simulink model "S_Mod_Sim_PV_V1"  (R2017a)
settings: Solver=VariableStepAuto  StartTime=0.0  StopTime=1.3  FixedStep=1e-6  MaxStep=1e-4  RelTol=1e-3
values from neighbouring files (symbols this model uses):
  Cdc = 470e-6    (= 0.00047)    [M_Mod_Sim_PV_V1.m]
  Cin = 1e-6    (= 1e-06)    [M_Mod_Sim_PV_V1.m]
  dIL = (vpv/L)*d*Ts1    (= 0.460350492963)    [M_Mod_Sim_PV_V1.m]
  Fred = fs    (= 60)    [M_Mod_Sim_PV_V1.m]
  fs = 60    [M_Mod_Sim_PV_V1.m]
  Icc_calc = In/(5/100)    [M_Mod_Sim_PV_V1.m]
  Kf1 = Scala/dDmax    (= 5.88235294118)    [M_Mod_Sim_PV_V1.m]
  ki = 1/ipv    (= 0.0636345580933)    [M_Mod_Sim_PV_V1.m]
  KI2 = Ki2*Ts4    [M_Mod_Sim_PV_V1.m]
  KI4 = Ki4*Ts4    [M_Mod_Sim_PV_V1.m]
  KI5 = Ki5*Ts_inv    (= 0.0710611516878)    [M_Mod_Sim_PV_V1.m]
  KP2 = Kp2 - KI2/2    [M_Mod_Sim_PV_V1.m]
  KP4 = Kp4 - KI4/2    [M_Mod_Sim_PV_V1.m]
  KP5 = Kp5*Ts_inv - KI5/2    (= -0.0349975104025)    [M_Mod_Sim_PV_V1.m]
  L = 68.2729*Lmin    (= 0.100000049318)    [M_Mod_Sim_PV_V1.m]
  Linv = 0.035    [M_Mod_Sim_PV_V1.m]
  Rinv = 0.0417    [M_Mod_Sim_PV_V1.m]
  S = 10e3*3/2    (= 15000)    [M_Mod_Sim_PV_V1.m]
  Ts1 = 1/Fs    (= 0.0002)    [M_Mod_Sim_PV_V1.m]
  Ts3 = Ts1    (= 0.0002)    [M_Mod_Sim_PV_V1.m]
  Ts4 = 1/(4*Fc)    (= 5e-05)    [M_Mod_Sim_PV_V1.m]
  Ts_inv = 1/(100*Fc)    (= 2e-06)    [M_Mod_Sim_PV_V1.m]
  vdc = 1000    [M_Mod_Sim_PV_V1.m]
  vdc_ref = vdc    (= 1000)    [M_Mod_Sim_PV_V1.m]
  Vf = VL/sqrt(3)    [M_Mod_Sim_PV_V1.m]
  VL = (381.051/2)    (= 190.5255)    [M_Mod_Sim_PV_V1.m]
undefined symbols (not defined in the file or in its folder): DiscIntNeverNeededParam
undefined symbols (not defined in the file): Fs
libraries: powerlib x15, powerlib_meascontrol x12, fuzblock x3, dsparch4 x3, re_lib x1
settings Model: Creator=dricl  LastModifiedBy=dricl

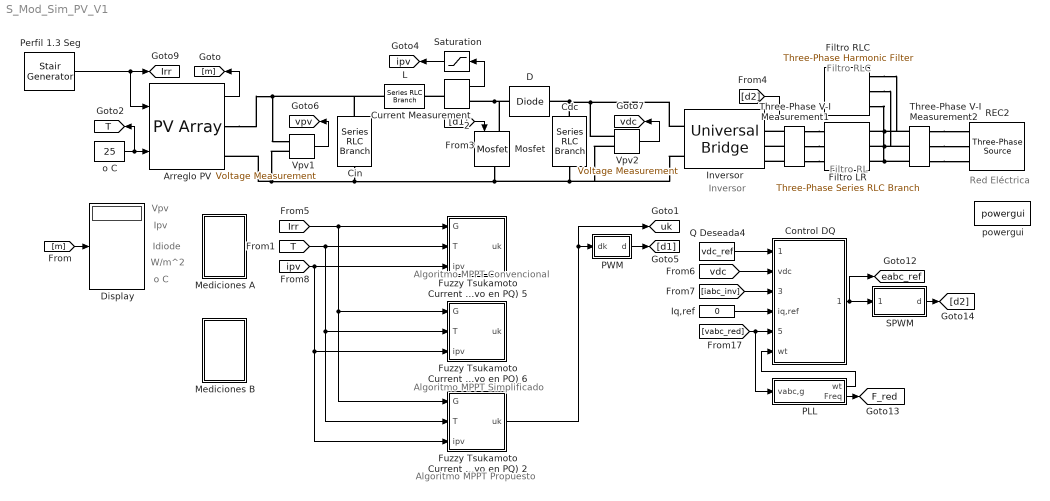
== system S_Mod_Sim_PV_V1 ==
  note: o C
  note: Idiode
  note: Ipv
  note: Vpv
  note: W/m^2
  note: Red Eléctrica
  note: Filtro RL
  note: Inversor
  note: Filtro RLC
  note: Algoritmo MPPT Convencional
  note: Algoritmo MPPT Simplificado
  note: Algoritmo MPPT Propuesto
  " Control DQ" : Subsystem
  Arreglo PV : re_lib/Solar/PV Array  Npar=No_Cadenas_Paralelo  Nser=No_Modulos_PorCadena  PlotType=array @ 1000 W/m2 & specified temperatures  S_vec=[ 1250 1000 100 ]  Temp_C_vec="[ 45 25  0]"  ModuleName=Canadian Solar CS6X-280P  PlotWhenSelected=off  Pm=279.816  Ncell=72  Voc=44.2  Isc=8.42  Vm=35.6  Im=7.86  beta_Voc_pc=-0.39  alpha_Isc_pc=0.06  beta_Voc=-0.17238  alpha_Isc=0.005052  IL=8.4417  I0=7.7188e-10  nI=1.0345  Rsh=300.2269  Rs=0.38773  BAL=off  Tc=1e-6  Tfilter=5e-5
  Cdc : powerlib/Elements/Series RLC Branch  LConnTagsString=__new0  RConnTagsString=__new0  BranchType=C  Resistance=0.01  Inductance=1e-3  SetiL0=off  InitialCurrent=0  Capacitance=Cdc  Setx0=on  InitialVoltage=vdc_ref  Measurements=None
  Cin : powerlib/Elements/Series RLC Branch  LConnTagsString=__new0  RConnTagsString=__new0  BranchType=C  Resistance=0.01  Inductance=1e-3  SetiL0=off  InitialCurrent=0  Capacitance=Cin  Setx0=off  InitialVoltage=640.8  Measurements=None
  Current Measurement2 : powerlib/Measurements/Current Measurement  PhasorSimulation=off  OutputType=Complex  PSBequivalent=0
  D : powerlib/Power Electronics/Diode  Ron=0.001  Lon=0  Vf=0  IC=0  UseSnubber=0  Rs=500  Cs=250e-9  Measurements=off
  Display : Display
  Filtro LR : powerlib/Elements/Three-Phase Series RLC Branch  LConnTagsString=A|B|C  RConnTagsString=A|B|C  BranchType=RL  Resistance=Rinv  Inductance=Linv  Capacitance=1e-6  Measurements=None
  Filtro RLC : powerlib/Elements/Three-Phase Harmonic Filter  LConnTagsString=A|B|C  FilterType=Single-tuned  FilterConnection=Y (grounded)  ParNom=[VL fs]  Qc=S*0.001  Fr=[31.42*60]  Frd=[40*fs 80*fs]  Q=5  Measurements=None
      settings: AttributesFormatString=\n  SourceProductName=Simscape Power Systems  SourceProductBaseCode=PS
  "Fuzzy Tsukamoto Current Controller n_mppt = 99.11%, ta(2%) = 0.12 s con Steps de Irrad Interv. 2 Seg. n_mppt = 96.74%, ta(2%) = 0.12 s con Steps de Irrad Interv. 0.5 Seg. n_mppt = 99.37%, ta(2%) = 0.12 s con Curva de Irrad Este controlador puede disminuir ta e incrementar a tr para mitigar los MP en id (impacto positivo en PQ) 2" : Subsystem
  "Fuzzy Tsukamoto Current Controller n_mppt = 99.11%, ta(2%) = 0.12 s con Steps de Irrad Interv. 2 Seg. n_mppt = 96.74%, ta(2%) = 0.12 s con Steps de Irrad Interv. 0.5 Seg. n_mppt = 99.37%, ta(2%) = 0.12 s con Curva de Irrad Este controlador puede disminuir ta e incrementar a tr para mitigar los MP en id (impacto positivo en PQ) 5" : Subsystem
  "Fuzzy Tsukamoto Current Controller n_mppt = 99.11%, ta(2%) = 0.12 s con Steps de Irrad Interv. 2 Seg. n_mppt = 96.74%, ta(2%) = 0.12 s con Steps de Irrad Interv. 0.5 Seg. n_mppt = 99.37%, ta(2%) = 0.12 s con Curva de Irrad Este controlador puede disminuir ta e incrementar a tr para mitigar los MP en id (impacto positivo en PQ) 6" : Subsystem
  Inversor : powerlib/Power Electronics/Universal Bridge  Arms=3  SnubberResistance=1e5  SnubberCapacitance=inf  Device=IGBT / Diodes  Ron=1e-3  Lon=0  ForwardVoltages="[  0  0  ]"  ForwardVoltage=0  GTOparameters=[ 10e-6 , 20e-6 ]  IGBTparameters=[ 1e-6 , 2e-6 ]  Measurements=None  Measurements_2=None  converterType=Rectifier
  Iq,ref : Constant  Value=0  SampleTime=Ts4
  L : powerlib/Elements/Series RLC Branch  LConnTagsString=__new0  RConnTagsString=__new0  BranchType=L  Resistance=40.76340  Inductance=L  SetiL0=off  InitialCurrent=0  Capacitance=1e-6  Setx0=off  InitialVoltage=0  Measurements=None
  Mediciones A : Subsystem
  Mediciones B : Subsystem
  Mosfet : powerlib/Power Electronics/Mosfet  Ron=0.001  Lon=0  Rd=0  Vfd=0  IC=0  Rs=1e5  Cs=inf  Measurements=off
  PLL : Subsystem
  PWM : Subsystem  AncestorBlock=plecslib_extras2/Modulators/Symmetrical PWM  mask(Symmetrical PWM){sampling=Natural (carrier starts with 0), fc=Fs, offset=0, input_limits=[0 Kf1], output_values=[0 1]}
      mask prompts: fc "Carrier frequency (Hz):"; offset "Carrier offset (p.u.):"; input_limits "Input limits [min max]:"; output_values "Output values [off on]:"
      mask help: PWM generator with a symmetrical triangular carrier. If the input is a vector, the output is also a vector of the same width.
      mask init:
      | if numel(fc)>1 || fc<=0,
      |   error('Carrier frequency must be a positive scalar.');
      | end
      | if numel(offset)>1 || offset<0 || offset>=1,
      |   error('Carrier offset must be a scalar in the range [0; 1/fc[.');
      | end
      | if sampling == 1,
      |   offset = mod(offset+.75, 1);
      | end
      | 
      | si = [.5 mod(offset, .5)]/fc;
      mask Help: eval('plecs(''help'', ''symmetricalpwm.html'')')
      mask TypeOptions sampling: Natural (carrier starts with 0) | Natural (carrier starts with 1) | Regular (double edge) | Regular (single edge)
  Perfil 1.3 Seg : powerlib_meascontrol/Pulse & Signal Generators/Stair Generator  t=[0, 0.1, 0.3, 0.5, 0.7, 0.9, 1.1]  e=[0, 1000, 400, 800, 500, 900, 600]  Ts=0
      settings: SourceProductName=Simscape Power Systems
  Q Deseada4 : Constant  Value=vdc_ref  SampleTime=Ts4
  REC2 : powerlib/Electrical Sources/Three-Phase Source  InternalConnection=Yg  VoltagePhases=on  Voltage=VL  PhaseAngle=0  Voltage_phases=[VL/sqrt(3) VL/sqrt(3) VL/sqrt(3)]  PhaseAngles_phases=[0 -120 +120]  Frequency=Fred  NonIdealSource=on  SpecifyImpedance=on  Resistance=25e3^2/10e6/5  Inductance=25e3^2/10e6/377  ShortCircuitLevel=Icc_calc*2  BaseVoltage=VL  XRratio=7  BusType=swing  Pref=-500e3  Qref=0  Prefabc=[10e3, 10e3, 10e3]  Qrefabc=[0, 0, 0]  Qmin=-inf  Qmax=inf
  SPWM : Subsystem
  Saturation : Saturate  UpperLimit=inf  LowerLimit=0
  Three-Phase V-I Measurement1 : powerlib/Measurements/Three-Phase V-I Measurement  VoltageMeasurement=phase-to-ground  SetLabelV=on  LabelV=vabc_inv  Vpu=off  VpuLL=off  CurrentMeasurement=yes  SetLabelI=on  LabelI=iabc_inv  Ipu=off  Pbase=100e6  Vbase=500e3  OutputType=Complex  PhasorSimulation=off  PSBequivalent=0
  Three-Phase V-I Measurement2 : powerlib/Measurements/Three-Phase V-I Measurement  VoltageMeasurement=phase-to-ground  SetLabelV=on  LabelV=vabc_red  Vpu=off  VpuLL=off  CurrentMeasurement=yes  SetLabelI=on  LabelI=iabc_red  Ipu=off  Pbase=100e6  Vbase=500e3  OutputType=Complex  PhasorSimulation=off  PSBequivalent=0
  Vpv1 : powerlib/Measurements/Voltage Measurement  PhasorSimulation=off  OutputType=Complex  PSBequivalent=0
  Vpv2 : powerlib/Measurements/Voltage Measurement  PhasorSimulation=off  OutputType=Complex  PSBequivalent=0
  o C : Constant  Value=25
  powergui : powerlib/powergui  Priority=1  SimulationMode=Continuous  SampleTime=1e-6  frequency=60  Iterations=50  frequencyindice=0  Pbase=100e6  ErrMax=1e-4  UnitsV=kV  UnitsW=MW  buscounter=0  FunctionMessages=off  echomessages=off  EnableUseOfTLC=off  CurrentSourceSwitches=off  DisableSnubberDevices=off  DisableRonSwitches=off  DisableVfSwitches=off  DisplayEquations=off  SolverType=Tustin/Backward Euler (TBE)  Interpol=off  ExternalGateDelay=off  methode=off  Ts=100  x0status=blocks  SPID=on  SwTol=0  HookPort=off  RestoreLinks=warning  ResistiveCurrentMeasurement=off  Frange=[0:2:500]  Ylog=off  Xlog=on  ShowGrid=off  save=off  variable=ZData  structure=logsout  ZoomFFT=on  StartTime=0.1  cycles=4  DisplayStyle=1  fundamental=60  FreqAxis=off  MaxFrequency=1000  frequencyindicesteady=1  RmsSteady=1  display=off
  tag scope: F_red=global, Irr=global, T=global, eabc_ref=global, ipv=global, uk=global, vdc=global, vpv=global
  wires:
  o C/1 -> [T], Arreglo PV/2
  Arreglo PV/1 -> [m]
  [m] -> Display/1
  Current Measurement2/1 -> Saturation/1
  Vpv1/1 -> [vpv]
  Vpv2/1 -> [vdc]
  [d1] -> Mosfet/1
  [d2] -> Inversor/1
  [vabc_red] -> " Control DQ"/5(vabc,red), PLL/1(vabc,g)
  PLL/1(wt) -> " Control DQ"/6(wt)
  [iabc_inv] -> " Control DQ"/3(iabc,inv)
  " Control DQ"/1(eabc,ref) -> [eabc_ref], SPWM/1(eabc,ref)
  PLL/2(Freq) -> [F_red]
  Iq,ref/1 -> " Control DQ"/4(iq,ref)
  [vdc] -> " Control DQ"/2(vdc)
  SPWM/1(d) -> [d2]
  PWM/1(d) -> [d1]
  Saturation/1 -> [ipv]
  Q Deseada4/1 -> " Control DQ"/1(vdc,ref)
  Perfil 1.3 Seg/1 -> Arreglo PV/1, [Irr]
  [Irr] -> "Fuzzy Tsukamoto Current Controller n_mppt = 99.11%, ta(2%) = 0.12 s con Steps de Irrad Interv. 2 Seg. n_mppt = 96.74%, ta(2%) = 0.12 s con Steps de Irrad Interv. 0.5 Seg. n_mppt = 99.37%, ta(2%) = 0.12 s con Curva de Irrad Este controlador puede disminuir ta e incrementar a tr para mitigar los MP en id (impacto positivo en PQ) 2"/1(G), "Fuzzy Tsukamoto Current Controller n_mppt = 99.11%, ta(2%) = 0.12 s con Steps de Irrad Interv. 2 Seg. n_mppt = 96.74%, ta(2%) = 0.12 s con Steps de Irrad Interv. 0.5 Seg. n_mppt = 99.37%, ta(2%) = 0.12 s con Curva de Irrad Este controlador puede disminuir ta e incrementar a tr para mitigar los MP en id (impacto positivo en PQ) 6"/1(G), "Fuzzy Tsukamoto Current Controller n_mppt = 99.11%, ta(2%) = 0.12 s con Steps de Irrad Interv. 2 Seg. n_mppt = 96.74%, ta(2%) = 0.12 s con Steps de Irrad Interv. 0.5 Seg. n_mppt = 99.37%, ta(2%) = 0.12 s con Curva de Irrad Este controlador puede disminuir ta e incrementar a tr para mitigar los MP en id (impacto positivo en PQ) 5"/1(G)
  [ipv] -> "Fuzzy Tsukamoto Current Controller n_mppt = 99.11%, ta(2%) = 0.12 s con Steps de Irrad Interv. 2 Seg. n_mppt = 96.74%, ta(2%) = 0.12 s con Steps de Irrad Interv. 0.5 Seg. n_mppt = 99.37%, ta(2%) = 0.12 s con Curva de Irrad Este controlador puede disminuir ta e incrementar a tr para mitigar los MP en id (impacto positivo en PQ) 5"/3(ipv), "Fuzzy Tsukamoto Current Controller n_mppt = 99.11%, ta(2%) = 0.12 s con Steps de Irrad Interv. 2 Seg. n_mppt = 96.74%, ta(2%) = 0.12 s con Steps de Irrad Interv. 0.5 Seg. n_mppt = 99.37%, ta(2%) = 0.12 s con Curva de Irrad Este controlador puede disminuir ta e incrementar a tr para mitigar los MP en id (impacto positivo en PQ) 2"/3(ipv), "Fuzzy Tsukamoto Current Controller n_mppt = 99.11%, ta(2%) = 0.12 s con Steps de Irrad Interv. 2 Seg. n_mppt = 96.74%, ta(2%) = 0.12 s con Steps de Irrad Interv. 0.5 Seg. n_mppt = 99.37%, ta(2%) = 0.12 s con Curva de Irrad Este controlador puede disminuir ta e incrementar a tr para mitigar los MP en id (impacto positivo en PQ) 6"/3(ipv)
  [T] -> "Fuzzy Tsukamoto Current Controller n_mppt = 99.11%, ta(2%) = 0.12 s con Steps de Irrad Interv. 2 Seg. n_mppt = 96.74%, ta(2%) = 0.12 s con Steps de Irrad Interv. 0.5 Seg. n_mppt = 99.37%, ta(2%) = 0.12 s con Curva de Irrad Este controlador puede disminuir ta e incrementar a tr para mitigar los MP en id (impacto positivo en PQ) 2"/2(T), "Fuzzy Tsukamoto Current Controller n_mppt = 99.11%, ta(2%) = 0.12 s con Steps de Irrad Interv. 2 Seg. n_mppt = 96.74%, ta(2%) = 0.12 s con Steps de Irrad Interv. 0.5 Seg. n_mppt = 99.37%, ta(2%) = 0.12 s con Curva de Irrad Este controlador puede disminuir ta e incrementar a tr para mitigar los MP en id (impacto positivo en PQ) 6"/2(T), "Fuzzy Tsukamoto Current Controller n_mppt = 99.11%, ta(2%) = 0.12 s con Steps de Irrad Interv. 2 Seg. n_mppt = 96.74%, ta(2%) = 0.12 s con Steps de Irrad Interv. 0.5 Seg. n_mppt = 99.37%, ta(2%) = 0.12 s con Curva de Irrad Este controlador puede disminuir ta e incrementar a tr para mitigar los MP en id (impacto positivo en PQ) 5"/2(T)
  "Fuzzy Tsukamoto Current Controller n_mppt = 99.11%, ta(2%) = 0.12 s con Steps de Irrad Interv. 2 Seg. n_mppt = 96.74%, ta(2%) = 0.12 s con Steps de Irrad Interv. 0.5 Seg. n_mppt = 99.37%, ta(2%) = 0.12 s con Curva de Irrad Este controlador puede disminuir ta e incrementar a tr para mitigar los MP en id (impacto positivo en PQ) 2"/1(uk) -> [uk], PWM/1(dk)
  connections:
  Arreglo PV/RConn1 -- Cin/LConn1 -- L/LConn1 -- Vpv1/LConn1
  Current Measurement2/LConn1 -- L/RConn1
  Mosfet/LConn1 -- D/LConn1 -- Current Measurement2/RConn1
  Vpv2/LConn1 -- Inversor/RConn1 -- Cdc/LConn1 -- D/RConn1
  Vpv1/LConn2 -- Cin/RConn1 -- Vpv2/LConn2 -- Inversor/RConn2 -- Cdc/RConn1 -- Mosfet/RConn1 -- Arreglo PV/RConn2
  Three-Phase V-I Measurement2/RConn1 -- REC2/RConn1
  Three-Phase V-I Measurement2/RConn2 -- REC2/RConn2
  Three-Phase V-I Measurement2/RConn3 -- REC2/RConn3
  Filtro LR/RConn2 -- Three-Phase V-I Measurement2/LConn2 -- Filtro RLC/LConn2
  Filtro LR/RConn3 -- Three-Phase V-I Measurement2/LConn3 -- Filtro RLC/LConn3
  Filtro LR/RConn1 -- Three-Phase V-I Measurement2/LConn1 -- Filtro RLC/LConn1
  Three-Phase V-I Measurement1/RConn1 -- Filtro LR/LConn1
  Three-Phase V-I Measurement1/LConn1 -- Inversor/LConn1
  Three-Phase V-I Measurement1/RConn3 -- Filtro LR/LConn3
  Three-Phase V-I Measurement1/LConn3 -- Inversor/LConn3
  Three-Phase V-I Measurement1/RConn2 -- Filtro LR/LConn2
  Three-Phase V-I Measurement1/LConn2 -- Inversor/LConn2

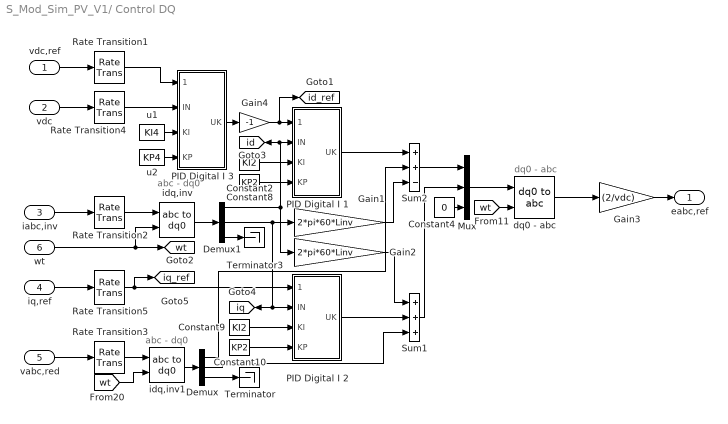
== system S_Mod_Sim_PV_V1/ Control DQ ==
  note: dq0 - abc
  note: abc - dq0
  note: abc - dq0
  vdc,ref : Inport
  vdc : Inport  Port=2
  iabc,inv : Inport  Port=3
  iq,ref : Inport  Port=4
  vabc,red : Inport  Port=5
  wt : Inport  Port=6
  Constant10 : Constant  Value=KP2  SampleTime=Ts4
  Constant2 : Constant  Value=KI2  SampleTime=Ts4
  Constant4 : Constant  Value=0  SampleTime=Ts4
  Constant8 : Constant  Value=KP2  SampleTime=Ts4
  Constant9 : Constant  Value=KI2  SampleTime=Ts4
  Demux : Demux  Outputs=3
  Demux1 : Demux  Outputs=3
  Gain1 : Gain  Gain=2*pi*60*Linv
  Gain2 : Gain  Gain=2*pi*60*Linv
  Gain3 : Gain  Gain=(2/vdc)
  Gain4 : Gain  Gain=-1
  Mux : Mux  Inputs=3
  PID Digital I 1 : MATLAB Function  TreatAsAtomicUnit=on
  PID Digital I 2 : MATLAB Function  TreatAsAtomicUnit=on
  PID Digital I 3 : MATLAB Function  TreatAsAtomicUnit=on
  Rate Transition{1..5} (5 alike) : RateTransition  OutPortSampleTime=Ts4
  Sum1 : Sum  Inputs=+++
  Sum2 : Sum  Inputs=++-
  Terminator : Terminator
  Terminator3 : Terminator
  dq0 - abc : powerlib_meascontrol/Transformations/dq0 to abc  Alignment=90 degrees behind phase A axis
  idq,inv : powerlib_meascontrol/Transformations/abc to dq0  Alignment=90 degrees behind phase A axis
  idq,inv1 : powerlib_meascontrol/Transformations/abc to dq0  Alignment=90 degrees behind phase A axis
  u1 : Constant  Value=KI4  SampleTime=Ts4
  u2 : Constant  Value=KP4  SampleTime=Ts4
  eabc,ref : Outport
  tag scope: id=global, id_ref=global, iq=global, iq_ref=global, wt=global
  wires:
  vabc,red/1 -> Rate Transition3/1
  Rate Transition4/1 -> PID Digital I 3/2(IN)
  Demux/2 -> Sum1/3
  Demux1/2 -> PID Digital I 2/2(IN), [iq], Gain1/1
  PID Digital I 1/1(UK) -> Sum2/1
  Gain4/1 -> [id_ref], PID Digital I 1/1(IN_ref)
  Sum1/1 -> Mux/2
  Mux/1 -> dq0 - abc/1
  Constant4/1 -> Mux/3
  [wt] -> dq0 - abc/2
  Demux/3 -> Terminator/1
  Demux1/1 -> [id], PID Digital I 1/2(IN), Gain2/1
  Constant8/1 -> PID Digital I 1/4(KP)
  Rate Transition5/1 -> [iq_ref], PID Digital I 2/1(IN_ref)
  idq,inv1/1 -> Demux/1
  iq,ref/1 -> Rate Transition5/1
  idq,inv/1 -> Demux1/1
  Constant9/1 -> PID Digital I 2/3(KI)
  u1/1 -> PID Digital I 3/3(KI)
  vdc,ref/1 -> Rate Transition1/1
  Constant10/1 -> PID Digital I 2/4(KP)
  vdc/1 -> Rate Transition4/1
  Constant2/1 -> PID Digital I 1/3(KI)
  iabc,inv/1 -> Rate Transition2/1
  Rate Transition2/1 -> idq,inv/1
  Demux1/3 -> Terminator3/1
  Rate Transition3/1 -> idq,inv1/1
  u2/1 -> PID Digital I 3/4(KP)
  PID Digital I 2/1(UK) -> Sum1/2
  Sum2/1 -> Mux/1
  Demux/1 -> Sum2/2
  Gain2/1 -> Sum1/1
  Gain1/1 -> Sum2/3
  [wt] -> idq,inv1/2
  wt/1 -> [wt], idq,inv/2
  dq0 - abc/1 -> Gain3/1
  PID Digital I 3/1(UK) -> Gain4/1
  Rate Transition1/1 -> PID Digital I 3/1(IN_ref)
  Gain3/1 -> eabc,ref/1

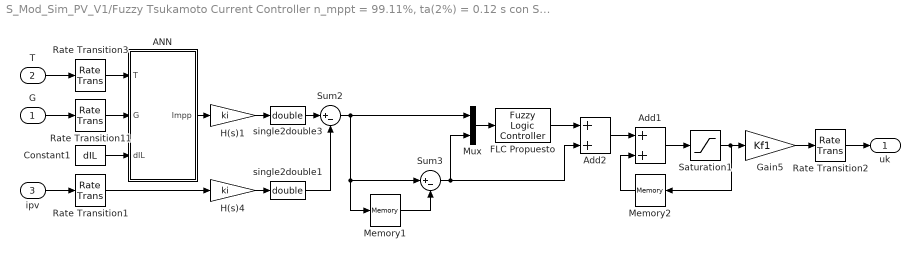
== system S_Mod_Sim_PV_V1/Fuzzy Tsukamoto Current Controller n_mppt = 99.11%, ta(2%) = 0.12 s con Steps de Irrad Interv. 2 Seg. n_mppt = 96.74%, ta(2%) = 0.12 s con Steps de Irrad Interv. 0.5 Seg. n_mppt = 99.37%, ta(2%) = 0.12 s con Curva de Irrad Este controlador puede disminuir ta e incrementar a tr para mitigar los MP en id (impacto positivo en PQ) 2 ==
  G : Inport
  T : Inport  Port=2
  ipv : Inport  Port=3
  ANN : MATLAB Function  TreatAsAtomicUnit=on
  Add1 : Sum
  Add2 : Sum
  Constant1 : Constant  Value=dIL  SampleTime=Ts3
  FLC Propuesto : fuzblock/Fuzzy Logic  Controller  fis=['5_Rules_MaMPPTCtrl_V1.fis']
  Gain5 : Gain  Gain=Kf1
  H(s)1 : Gain  Gain=ki
  H(s)4 : Gain  Gain=ki
  Memory1 : Memory  InheritSampleTime=on
  Memory2 : Memory  InheritSampleTime=on
  Mux : Mux  Inputs=2
  Rate Transition{1..3,11} (4 alike) : RateTransition  Deterministic=off  OutPortSampleTime=Ts3
  Saturation1 : Saturate  UpperLimit=1  LowerLimit=0
  Sum2 : Sum  Inputs=|+-
  Sum3 : Sum  Inputs=|+-
  single2double1 : DataTypeConversion  OutDataTypeStr=double
  single2double3 : DataTypeConversion  OutDataTypeStr=double
  uk : Outport
  wires:
  Rate Transition2/1 -> uk/1
  Memory2/1 -> Add1/2
  single2double3/1 -> Sum2/1
  single2double1/1 -> Sum2/2
  Memory1/1 -> Sum3/2
  Add1/1 -> Saturation1/1
  Saturation1/1 -> Memory2/1, Gain5/1
  Gain5/1 -> Rate Transition2/1
  H(s)1/1 -> single2double3/1
  H(s)4/1 -> single2double1/1
  ANN/1(Impp) -> H(s)1/1
  Mux/1 -> FLC Propuesto/1
  Sum2/1 -> Memory1/1, Sum3/1, Mux/1
  Sum3/1 -> Add2/2, Mux/2
  FLC Propuesto/1 -> Add2/1
  Add2/1 -> Add1/1
  G/1 -> Rate Transition11/1
  ipv/1 -> Rate Transition1/1
  Rate Transition1/1 -> H(s)4/1
  Rate Transition3/1 -> ANN/1(T)
  Rate Transition11/1 -> ANN/2(G)
  Constant1/1 -> ANN/3(dIL)
  T/1 -> Rate Transition3/1

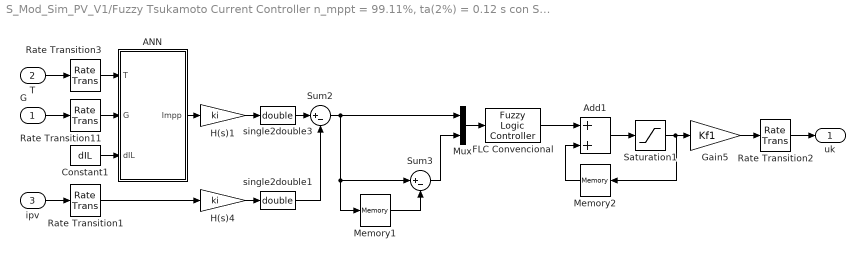
== system S_Mod_Sim_PV_V1/Fuzzy Tsukamoto Current Controller n_mppt = 99.11%, ta(2%) = 0.12 s con Steps de Irrad Interv. 2 Seg. n_mppt = 96.74%, ta(2%) = 0.12 s con Steps de Irrad Interv. 0.5 Seg. n_mppt = 99.37%, ta(2%) = 0.12 s con Curva de Irrad Este controlador puede disminuir ta e incrementar a tr para mitigar los MP en id (impacto positivo en PQ) 5 ==
  G : Inport
  T : Inport  Port=2
  ipv : Inport  Port=3
  ANN : MATLAB Function  TreatAsAtomicUnit=on
  Add1 : Sum
  Constant1 : Constant  Value=dIL  SampleTime=Ts3
  FLC Convencional : fuzblock/Fuzzy Logic  Controller  fis=['49_Rules_MaMPPTCtrlPaperShaikRAfi_V2.fis']
  Gain5 : Gain  Gain=Kf1
  H(s)1 : Gain  Gain=ki
  H(s)4 : Gain  Gain=ki
  Memory1 : Memory  InheritSampleTime=on
  Memory2 : Memory  InheritSampleTime=on
  Mux : Mux  Inputs=2
  Rate Transition{1..3,11} (4 alike) : RateTransition  Deterministic=off  OutPortSampleTime=Ts3
  Saturation1 : Saturate  UpperLimit=1  LowerLimit=0
  Sum2 : Sum  Inputs=|+-
  Sum3 : Sum  Inputs=|+-
  single2double1 : DataTypeConversion  OutDataTypeStr=double
  single2double3 : DataTypeConversion  OutDataTypeStr=double
  uk : Outport
  wires:
  Rate Transition2/1 -> uk/1
  Memory2/1 -> Add1/2
  single2double3/1 -> Sum2/1
  single2double1/1 -> Sum2/2
  Rate Transition1/1 -> H(s)4/1
  G/1 -> Rate Transition11/1
  ipv/1 -> Rate Transition1/1
  Memory1/1 -> Sum3/2
  Add1/1 -> Saturation1/1
  Saturation1/1 -> Memory2/1, Gain5/1
  Gain5/1 -> Rate Transition2/1
  H(s)1/1 -> single2double3/1
  H(s)4/1 -> single2double1/1
  ANN/1(Impp) -> H(s)1/1
  Constant1/1 -> ANN/3(dIL)
  Mux/1 -> FLC Convencional/1
  Sum2/1 -> Memory1/1, Sum3/1, Mux/1
  Sum3/1 -> Mux/2
  FLC Convencional/1 -> Add1/1
  Rate Transition11/1 -> ANN/2(G)
  Rate Transition3/1 -> ANN/1(T)
  T/1 -> Rate Transition3/1

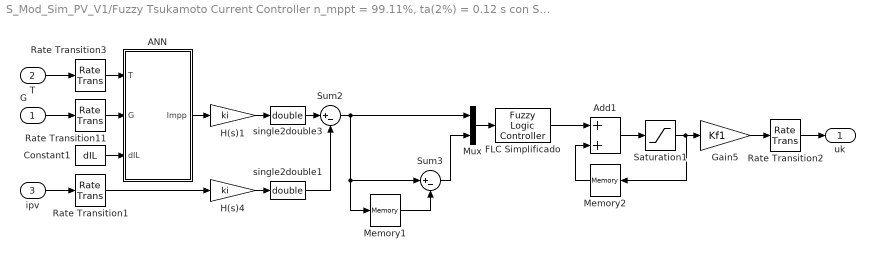
== system S_Mod_Sim_PV_V1/Fuzzy Tsukamoto Current Controller n_mppt = 99.11%, ta(2%) = 0.12 s con Steps de Irrad Interv. 2 Seg. n_mppt = 96.74%, ta(2%) = 0.12 s con Steps de Irrad Interv. 0.5 Seg. n_mppt = 99.37%, ta(2%) = 0.12 s con Curva de Irrad Este controlador puede disminuir ta e incrementar a tr para mitigar los MP en id (impacto positivo en PQ) 6 ==
  G : Inport
  T : Inport  Port=2
  ipv : Inport  Port=3
  ANN : MATLAB Function  TreatAsAtomicUnit=on
  Add1 : Sum
  Constant1 : Constant  Value=dIL  SampleTime=Ts3
  FLC Simplificado : fuzblock/Fuzzy Logic  Controller  fis=['5_Rules_MaMPPTCtrl_V1.fis']
  Gain5 : Gain  Gain=Kf1
  H(s)1 : Gain  Gain=ki
  H(s)4 : Gain  Gain=ki
  Memory1 : Memory  InheritSampleTime=on
  Memory2 : Memory  InheritSampleTime=on
  Mux : Mux  Inputs=2
  Rate Transition{1..3,11} (4 alike) : RateTransition  Deterministic=off  OutPortSampleTime=Ts3
  Saturation1 : Saturate  UpperLimit=1  LowerLimit=0
  Sum2 : Sum  Inputs=|+-
  Sum3 : Sum  Inputs=|+-
  single2double1 : DataTypeConversion  OutDataTypeStr=double
  single2double3 : DataTypeConversion  OutDataTypeStr=double
  uk : Outport
  wires:
  Rate Transition2/1 -> uk/1
  Memory2/1 -> Add1/2
  single2double3/1 -> Sum2/1
  single2double1/1 -> Sum2/2
  Rate Transition1/1 -> H(s)4/1
  ipv/1 -> Rate Transition1/1
  Memory1/1 -> Sum3/2
  Add1/1 -> Saturation1/1
  Saturation1/1 -> Memory2/1, Gain5/1
  Gain5/1 -> Rate Transition2/1
  H(s)1/1 -> single2double3/1
  H(s)4/1 -> single2double1/1
  Mux/1 -> FLC Simplificado/1
  Sum2/1 -> Memory1/1, Sum3/1, Mux/1
  Sum3/1 -> Mux/2
  FLC Simplificado/1 -> Add1/1
  Rate Transition11/1 -> ANN/2(G)
  Rate Transition3/1 -> ANN/1(T)
  G/1 -> Rate Transition11/1
  T/1 -> Rate Transition3/1
  Constant1/1 -> ANN/3(dIL)
  ANN/1(Impp) -> H(s)1/1

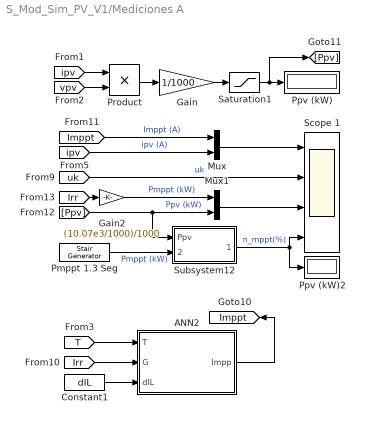
== system S_Mod_Sim_PV_V1/Mediciones A ==
  ANN2 : MATLAB Function  TreatAsAtomicUnit=on
  Constant1 : Constant  Value=dIL  SampleTime=Ts1
  Gain : Gain  Gain=1/1000
  Gain2 : Gain  Gain=(10.07e3/1000)/1000
  Mux : Mux  Inputs=2
  Mux1 : Mux  Inputs=2
  Pmppt 1.3 Seg : powerlib_meascontrol/Pulse & Signal Generators/Stair Generator  t=[0, 0.1, 0.3, 0.5, 0.7, 0.9, 1.1]  e=[0, 10.07, 4.040, 8.099, 5.066, 9.090, 6.086]*0.99755  Ts=0
      settings: SourceProductName=Simscape Power Systems
  Ppv (kW) : Display
  Ppv (kW)2 : Display
  Product : Product
  Saturation1 : Saturate  UpperLimit=inf  LowerLimit=0
  Scope 1 : Scope  NumInputPorts=4
  Subsystem12 : Subsystem
  tag scope: Imppt=global
  wires:
  [ipv] -> Product/1
  Product/1 -> Gain/1
  [vpv] -> Product/2
  Gain/1 -> Saturation1/1
  [Imppt] -> Mux/1  "Imppt (A)"
  [Ppv] -> Subsystem12/1(Ppv), Mux1/2  "Ppv (kW)"
  [ipv] -> Mux/2  "ipv (A)"
  [Irr] -> Gain2/1
  Gain2/1 -> Mux1/1  "Pmppt (kW)"
  [uk] -> Scope 1/2  "uk"
  Saturation1/1 -> [Ppv], Ppv (kW)/1
  Mux1/1 -> Scope 1/3
  Mux/1 -> Scope 1/1
  Pmppt 1.3 Seg/1 -> Subsystem12/2(Pmpp)  "Pmppt (kW)"
  Subsystem12/1(n_mppt) -> Scope 1/4, Ppv (kW)2/1  "n_mppt(%)"
  ANN2/1(Impp) -> [Imppt]
  Constant1/1 -> ANN2/3(dIL)
  [Irr] -> ANN2/2(G)
  [T] -> ANN2/1(T)

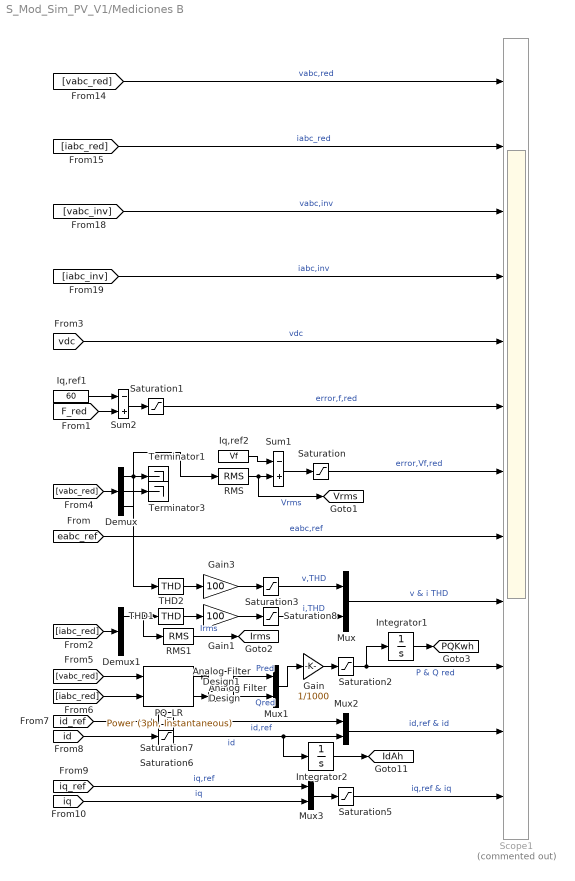
== system S_Mod_Sim_PV_V1/Mediciones B ==
  Analog Filter Design : dsparch4/Analog Filter Design  method=Butterworth  filttype=Lowpass  N=8  Wlo=4000  Whi=80  Rp=2  Rs=40
  Analog Filter Design1 : dsparch4/Analog Filter Design  method=Butterworth  filttype=Lowpass  N=8  Wlo=4000  Whi=80  Rp=2  Rs=40
  Demux : Demux  Outputs=3
  Demux1 : Demux  Outputs=3
  Gain : Gain  Gain=1/1000
  Gain1 : Gain  Gain=100
  Gain3 : Gain  Gain=100
  Integrator1 : Integrator  ZeroCross=off
  Integrator2 : Integrator  ZeroCross=off
  Iq,ref1 : Constant  Value=60  SampleTime=Ts4
  Iq,ref2 : Constant  Value=Vf  SampleTime=Ts4
  Mux{,1..3} (4 alike) : Mux  Inputs=2
  PQ_LR : powerlib_meascontrol/Measurements/Power (3ph, Instantaneous)
      settings: SourceProductName=Simscape Power Systems
  RMS : powerlib_meascontrol/Measurements/RMS  TrueRMS=on  Freq=60  RMSInit=0  Ts=0
  RMS1 : powerlib_meascontrol/Measurements/RMS  TrueRMS=on  Freq=60  RMSInit=0  Ts=0
  Saturation : Saturate  UpperLimit=5.5  LowerLimit=-5.5
  Saturation1 : Saturate  UpperLimit=1  LowerLimit=-1
  Saturation2 : Saturate  UpperLimit=20  LowerLimit=0
  Saturation3 : Saturate  UpperLimit=20  LowerLimit=0
  Saturation5 : Saturate  UpperLimit=100  LowerLimit=0
  Saturation6 : Saturate  UpperLimit=inf  LowerLimit=0
  Saturation7 : Saturate  UpperLimit=inf  LowerLimit=0
  Saturation8 : Saturate  UpperLimit=20  LowerLimit=0
  Scope1 : Scope  Commented=on  NumInputPorts=12
  Sum1 : Sum  Inputs=-+
  Sum2 : Sum  Inputs=-+
  THD1 : powerlib_meascontrol/Measurements/THD  Freq=60  Ts=0
  THD2 : powerlib_meascontrol/Measurements/THD  Freq=60  Ts=0
  Terminator1 : Terminator
  Terminator3 : Terminator
  tag scope: IdAh=global, Irms=global, PQKwh=global, Vrms=global
  wires:
  Saturation/1 -> Scope1/7  "error,Vf,red"
  [vabc_red] -> Scope1/1  "vabc,red"
  [eabc_ref] -> Scope1/8  "eabc,ref"
  [iabc_red] -> Scope1/2  "iabc_red"
  Demux/1 -> THD2/1, RMS/1
  [vdc] -> Scope1/5  "vdc"
  [iabc_inv] -> Scope1/4  "iabc,inv"
  [vabc_inv] -> Scope1/3  "vabc,inv"
  Sum1/1 -> Saturation/1
  RMS/1 -> [Vrms], Sum1/2  "Vrms"
  Demux/2 -> Terminator3/1
  Demux/3 -> Terminator1/1
  [vabc_red] -> Demux/1
  [F_red] -> Sum2/2
  Iq,ref2/1 -> Sum1/1
  Iq,ref1/1 -> Sum2/1
  Saturation1/1 -> Scope1/6  "error,f,red"
  Sum2/1 -> Saturation1/1
  [iabc_red] -> Demux1/1
  Demux1/1 -> RMS1/1, THD1/1
  THD2/1 -> Gain3/1
  THD1/1 -> Gain1/1
  Mux/1 -> Scope1/9  "v & i THD"
  [vabc_red] -> PQ_LR/1
  [iabc_red] -> PQ_LR/2
  PQ_LR/1 -> Analog Filter Design/1
  Analog Filter Design/1 -> Mux1/1  "Pred"
  PQ_LR/2 -> Analog Filter Design1/1
  Analog Filter Design1/1 -> Mux1/2  "Qred"
  Saturation2/1 -> Integrator1/1, Scope1/10  "P & Q red"
  Gain/1 -> Saturation2/1
  Mux1/1 -> Gain/1
  Mux3/1 -> Saturation5/1
  [iq] -> Mux3/2  "iq"
  [id] -> Saturation6/1
  [iq_ref] -> Mux3/1  "iq,ref"
  [id_ref] -> Saturation7/1
  Mux2/1 -> Scope1/11  "id,ref & id"
  Saturation5/1 -> Scope1/12  "iq,ref & iq"
  RMS1/1 -> [Irms]  "Irms"
  Saturation6/1 -> Integrator2/1, Mux2/2  "id"
  Saturation7/1 -> Mux2/1  "id,ref"
  Gain3/1 -> Saturation3/1
  Saturation3/1 -> Mux/1  "v,THD"
  Saturation8/1 -> Mux/2  "i,THD"
  Gain1/1 -> Saturation8/1
  Integrator2/1 -> [IdAh]
  Integrator1/1 -> [PQKwh]

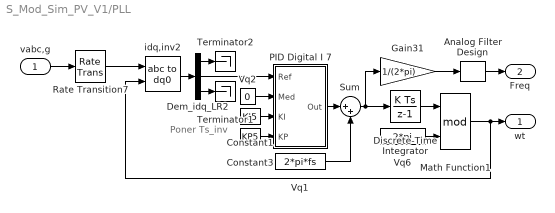
== system S_Mod_Sim_PV_V1/PLL ==
  note: Poner Ts_inv
  vabc,g : Inport
  Analog Filter Design : dsparch4/Analog Filter Design  method=Butterworth  filttype=Lowpass  N=8  Wlo=4000  Whi=80  Rp=2  Rs=40
  Constant1 : Constant  Value=KI5  SampleTime=Ts_inv
  Constant3 : Constant  Value=KP5  SampleTime=Ts_inv
  Dem_idq_LR2 : Demux  Outputs=3
  Discrete-Time Integrator : DiscreteIntegrator  InitialConditionSetting=State (most efficient)  SampleTime=Ts_inv  ICPrevOutput=DiscIntNeverNeededParam  ICPrevScaledInput=DiscIntNeverNeededParam
  Gain31 : Gain  Gain=1/(2*pi)  OutMin=[0.1]
  Math Function1 : Math  Operator=mod  SaturateOnIntegerOverflow=on
  PID Digital I 7 : MATLAB Function  TreatAsAtomicUnit=on
  Rate Transition7 : RateTransition  OutPortSampleTime=Ts_inv
  Sum : Sum  Inputs=|++
  Terminator1 : Terminator
  Terminator2 : Terminator
  Vq1 : Constant  Value=2*pi*fs  SampleTime=Ts_inv
  Vq2 : Constant  Value=0
  Vq6 : Constant  Value=2*pi  SampleTime=Ts_inv
  idq,inv2 : powerlib_meascontrol/Transformations/abc to dq0  Alignment=90 degrees behind phase A axis
  wt : Outport
  Freq : Outport  Port=2
  wires:
  Gain31/1 -> Analog Filter Design/1
  vabc,g/1 -> Rate Transition7/1
  idq,inv2/1 -> Dem_idq_LR2/1
  Vq6/1 -> Math Function1/2
  Discrete-Time Integrator/1 -> Math Function1/1
  Math Function1/1 -> wt/1, idq,inv2/2
  Vq2/1 -> PID Digital I 7/2(Med)
  Dem_idq_LR2/2 -> PID Digital I 7/1(Ref)
  Sum/1 -> Gain31/1, Discrete-Time Integrator/1
  Vq1/1 -> Sum/2
  PID Digital I 7/1(Out) -> Sum/1
  Constant1/1 -> PID Digital I 7/3(KI)
  Constant3/1 -> PID Digital I 7/4(KP)
  Dem_idq_LR2/3 -> Terminator1/1
  Dem_idq_LR2/1 -> Terminator2/1
  Rate Transition7/1 -> idq,inv2/1
  Analog Filter Design/1 -> Freq/1

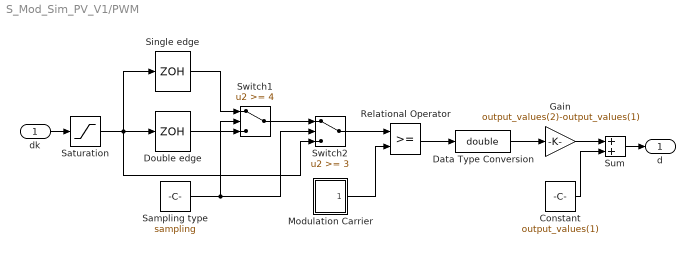
== system S_Mod_Sim_PV_V1/PWM ==
  dk : Inport
  Constant : Constant  Value=output_values(1)
  Data Type Conversion : DataTypeConversion  OutDataTypeStr=double  SaturateOnIntegerOverflow=on  RndMeth=Zero
  Double edge : ZeroOrderHold  SampleTime=si
  Gain : Gain  Gain=output_values(2)-output_values(1)  SaturateOnIntegerOverflow=on  OutDataTypeStr=Inherit: Same as input  ParamDataTypeStr=Inherit: Same as input
  Modulation Carrier : Subsystem  mask(Symmetric Triangle Generator){fc=fc, offset=mod(offset+.5, 1), range=input_limits}
      mask prompts: fc "Carrier frequency (Hz):"; offset "Carrier offset (p.u.):"; range "Signal range [min max]:"
      mask help: Generates a symmetrical triangular signal with output values between 0 and 1. The block forces the Simulink solver to output all tips of the signal. The output can therefore be used as a carrier signal for PWM.
      mask init:
      | if numel(fc)>1 || fc<=0,
      |   error('Carrier frequency must be a positive scalar.');
      | end
      | if numel(offset)>1 || offset<0 || offset>=1,
      |   error('Carrier offset must be a scalar in the interval [0; 1[.');
      | end
      | if numel(range)~=2,
      |   error('Signal range must be a two-element vector.')
      | end
      | if range(1)>=range(2),
      |   error('Signal range must be specified as [min max].')
      | end
      | 
      | carrier_t = [0 offset mod(1/2+offset, 1) 1]/fc;
      | carrier_v0 = 1-2*abs(offset-.5);
      | carrier_v = range(1)+[carrier_v0 0 1 carrier_v0]*diff(range);
      | [carrier_t, idx] = unique(carrier_t);
      | carrier_v = carrier_v(idx);
      | si = [.5 mod(offset, .5)]/fc;
      | 
      | L = length(carrier_t);
      | disp_seq_t = repmat(carrier_t(:),1,3) + ones(L,1)*[0,1,2]/fc;
      | disp_seq_v = repmat(carrier_v(:),1,3);
      mask Display: plot(disp_seq_t, disp_seq_v)
  Relational Operator : RelationalOperator  RndMeth=Nearest  InputSameDT=on
  Sampling type : Constant  Value=sampling
  Saturation : Saturate  UpperLimit=input_limits(2)  LowerLimit=input_limits(1)
  Single edge : ZeroOrderHold  SampleTime=[1 offset]/fc
  Sum : Sum  SaturateOnIntegerOverflow=on  InputSameDT=on  OutDataTypeStr=Inherit: Same as first input
  Switch1 : Switch  Threshold=4  SaturateOnIntegerOverflow=on  InputSameDT=on
  Switch2 : Switch  Threshold=3  SaturateOnIntegerOverflow=on  InputSameDT=on
  d : Outport
  wires:
  Data Type Conversion/1 -> Gain/1
  Constant/1 -> Sum/2
  Gain/1 -> Sum/1
  Sum/1 -> d/1
  Relational Operator/1 -> Data Type Conversion/1
  Switch2/1 -> Relational Operator/1
  Sampling type/1 -> Switch1/2, Switch2/2
  Single edge/1 -> Switch1/1
  Saturation/1 -> Double edge/1, Single edge/1, Switch2/3
  dk/1 -> Saturation/1
  Modulation Carrier/1(Out) -> Relational Operator/2
  Switch1/1 -> Switch2/1
  Double edge/1 -> Switch1/3

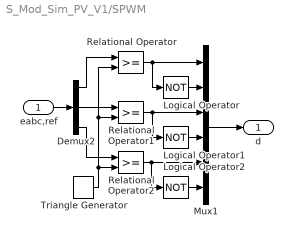
== system S_Mod_Sim_PV_V1/SPWM ==
  eabc,ref : Inport
  Demux2 : Demux  Outputs=3
  Logical Operator : Logic  Operator=NOT  AllPortsSameDT=off  OutDataTypeStr=boolean
  Logical Operator1 : Logic  Operator=NOT  AllPortsSameDT=off  OutDataTypeStr=boolean
  Logical Operator2 : Logic  Operator=NOT  AllPortsSameDT=off  OutDataTypeStr=boolean
  Mux1 : Mux  Inputs=6
  Relational Operator : RelationalOperator  OutDataTypeStr=boolean  RndMeth=Simplest
  Relational Operator1 : RelationalOperator  OutDataTypeStr=boolean  RndMeth=Simplest
  Relational Operator2 : RelationalOperator  OutDataTypeStr=boolean  RndMeth=Simplest
  Triangle Generator : powerlib_meascontrol/Pulse & Signal Generators/Triangle Generator  Freq=Fc  Phase=0  Ts=Ts_inv
  d : Outport
  wires:
  Logical Operator/1 -> Mux1/2
  Demux2/1 -> Relational Operator/1
  Demux2/2 -> Relational Operator1/1
  Logical Operator1/1 -> Mux1/4
  Relational Operator2/1 -> Mux1/5, Logical Operator2/1
  Triangle Generator/1 -> Relational Operator2/2, Relational Operator1/2, Relational Operator/2
  Mux1/1 -> d/1
  Relational Operator/1 -> Logical Operator/1, Mux1/1
  Logical Operator2/1 -> Mux1/6
  Demux2/3 -> Relational Operator2/1
  Relational Operator1/1 -> Logical Operator1/1, Mux1/3
  eabc,ref/1 -> Demux2/1

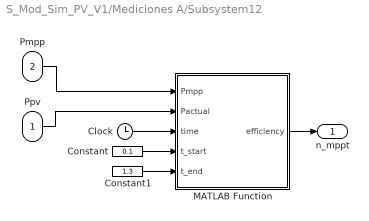
== system S_Mod_Sim_PV_V1/Mediciones A/Subsystem12 ==
  Ppv : Inport
  Pmpp : Inport  Port=2
  Clock : Clock
  Constant : Constant  Value=0.1
  Constant1 : Constant  Value=1.3
  MATLAB Function : MATLAB Function  TreatAsAtomicUnit=on
  n_mppt : Outport
  wires:
  MATLAB Function/1(efficiency) -> n_mppt/1
  Constant/1 -> MATLAB Function/4(t_start)
  Constant1/1 -> MATLAB Function/5(t_end)
  Pmpp/1 -> MATLAB Function/1(Pmpp)
  Ppv/1 -> MATLAB Function/2(Pactual)
  Clock/1 -> MATLAB Function/3(time)

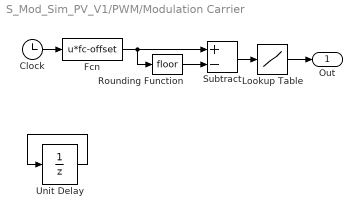
== system S_Mod_Sim_PV_V1/PWM/Modulation Carrier ==
  Clock : Clock
  Fcn : Fcn  Expr=u*fc-offset
  Lookup Table : Lookup  InputValues=[0 .5 1]  Table=[range(1) range(2) range(1)]  LookUpMeth=Interpolation-Use End Values
  Rounding Function : Rounding
  Subtract : Sum  Inputs=+-
  Unit Delay : UnitDelay  SampleTime=si
  Out : Outport
  wires:
  Lookup Table/1 -> Out/1
  Subtract/1 -> Lookup Table/1
  Rounding Function/1 -> Subtract/2
  Fcn/1 -> Rounding Function/1, Subtract/1
  Clock/1 -> Fcn/1
  Unit Delay/1 -> Unit Delay/1

== matlab function S_Mod_Sim_PV_V1/Mediciones A/ANN2 ==
  data: T input; G input; Impp output; dIL input
function Impp = ANN(T,G,dIL)

persistent w1 w2 b1 b2
persistent Media_T Media_G Media_Impp
persistent Std_T Std_G Std_Impp

if isempty(w1)

    data = load('ANN_parametros.mat');

    w1 = data.w1;
    w2 = data.w2;

    b1 = data.b1;
    b2 = data.b2;

    Media_T = data.Media_T;
    Media_G = data.Media_G;
    Media_Impp = data.Media_Impp;

    Std_T = data.Std_T;
    Std_G = data.Std_G;
    Std_Impp = data.Std_Impp;

end

%% =========================================================
% NORMALIZACION
% ==========================================================
% La red fue entrenada con:
%   x1 = T normalizada
%   x2 = G normalizada
%
% Por eso, antes de evaluar la ANN se aplica la misma
% normalización usada durante el entrenamiento.

x1 = (T - Media_T)/Std_T;
x2 = (G - Media_G)/Std_G;

%% =========================================================
% CAPA OCULTA
% ==========================================================
% Cada neurona oculta usa función logsig:
%
%   logsig(n) = 1/(1+exp(-n))

N1 = b1(1) + x1*w1(1,1) + x2*w1(1,2);
N1 = 1/(1+exp(-N1));

N2 = b1(2) + x1*w1(2,1) + x2*w1(2,2);
N2 = 1/(1+exp(-N2));

N3 = b1(3) + x1*w1(3,1) + x2*w1(3,2);
N3 = 1/(1+exp(-N3));

N4 = b1(4) + x1*w1(4,1) + x2*w1(4,2);
N4 = 1/(1+exp(-N4));

N5 = b1(5) + x1*w1(5,1) + x2*w1(5,2);
N5 = 1/(1+exp(-N5));

%% =========================================================
% CAPA DE SALIDA
% ==========================================================
% La salida de la red está normalizada.

Salida_norm = b2 + ...
              N1*w2(1,1) + ...
              N2*w2(1,2) + ...
              N3*w2(1,3) + ...
              N4*w2(1,4) + ...
              N5*w2(1,5);

%% =========================================================
% DESNORMALIZACION
% ==========================================================
% Se convierte la salida normalizada a amperes.

Impp_nom = Salida_norm*Std_Impp + Media_Impp;

%% =========================================================
% CORRECCION POR RIZO DE CORRIENTE dIL
% ==========================================================
% La ANN entrega una referencia nominal Impp_nom.
%
% dIL representa el rizo pico-a-pico de la corriente del inductor.
% Al restar dIL, la referencia se desplaza hacia abajo para evitar
% que la envolvente superior del rizo supere la corriente Impp.
%
% Esto es equivalente a:
%
%   Iref = Impp_nom - dIL
%
% Finalmente se satura a cero para evitar referencias negativas.

Impp = Impp_nom - dIL/2*1.13;

% Saturación inferior
Impp = max(Impp,0);

end

== matlab function S_Mod_Sim_PV_V1/ Control DQ/PID Digital I 1 ==
  data: IN_ref input; UK output; IN input; KI input; KP input
function UK = fcn(IN_ref, IN, KI, KP)

 %Valores iniciales de las conStantes del controlador
 persistent  ek uk
 persistent  ek_1 uk_1
 if isempty(ek)
    ek =0;
    uk =0;
    ek_1 =0;
    uk_1 =0;
 end
ek=IN_ref-IN;
uk=ek*(KP+KI)-ek_1*KP+uk_1;
if(uk>1000)
    uk=1000;
end
if(uk<-1000)
    uk=-1000;
end
ek_1=ek;
uk_1=uk;
UK=uk;
end

== matlab function S_Mod_Sim_PV_V1/ Control DQ/PID Digital I 2 ==
  data: IN_ref input; UK output; IN input; KI input; KP input
function UK = fcn(IN_ref, IN, KI, KP)

 %Valores iniciales de las conStantes del controlador
 persistent  ek uk
 persistent  ek_1 uk_1
 if isempty(ek)
    ek =0;
    uk =0;
    ek_1 =0;
    uk_1 =0;
 end
ek=IN_ref-IN;
uk=ek*(KP+KI)-ek_1*KP+uk_1;
if(uk>1000)
    uk=1000;
end
if(uk<-1000)
    uk=-1000;
end
ek_1=ek;
uk_1=uk;
UK=uk;
end

== matlab function S_Mod_Sim_PV_V1/ Control DQ/PID Digital I 3 ==
  data: IN_ref input; UK output; IN input; KI input; KP input
function UK = fcn(IN_ref, IN, KI, KP)

 %Valores iniciales de las conStantes del controlador
 persistent  ek uk
 persistent  ek_1 uk_1
 if isempty(ek)
    ek =0;
    uk =0;
    ek_1 =0;
    uk_1 =0;
 end
ek=IN_ref-IN;
uk=ek*(KP+KI)-ek_1*KP+uk_1;
if(uk>60)
    uk=60;
end
if(uk<-60)
    uk=-60;
end
ek_1=ek;
uk_1=uk;
UK=uk;
end

== matlab function S_Mod_Sim_PV_V1/PLL/PID Digital I 7 ==
  data: Ref input; Out output; Med input; KI input; KP input
function Out = fcn(Ref, Med, KI, KP)

 %Valores iniciales de las conStantes del controlador
 persistent  ek uk
 persistent  ek_1 uk_1
 if isempty(ek)
    ek =0;
    uk =0;
    ek_1 =0;
    uk_1 =0;
 end
ek=Ref-Med;
%uk=ek*(KP+KI)-ek_1*KP+uk_1;
uk=KP*ek+KI*ek+KI*ek_1;
ek_1=ek;
uk_1=uk;
Out=uk;
end

== matlab function S_Mod_Sim_PV_V1/Fuzzy Tsukamoto Current Controller n_mppt = 99.11%, ta(2%) = 0.12 s con Steps de Irrad Interv. 2 Seg. n_mppt = 96.74%, ta(2%) = 0.12 s con Steps de Irrad Interv. 0.5 Seg. n_mppt = 99.37%, ta(2%) = 0.12 s con Curva de Irrad Este controlador puede disminuir ta e incrementar a tr para mitigar los MP en id (impacto positivo en PQ) 2/ANN ==
  data: T input; G input; Impp output; dIL input
function Impp = ANN(T,G,dIL)

persistent w1 w2 b1 b2
persistent Media_T Media_G Media_Impp
persistent Std_T Std_G Std_Impp

if isempty(w1)

    data = load('ANN_parametros.mat');

    w1 = data.w1;
    w2 = data.w2;

    b1 = data.b1;
    b2 = data.b2;

    Media_T = data.Media_T;
    Media_G = data.Media_G;
    Media_Impp = data.Media_Impp;

    Std_T = data.Std_T;
    Std_G = data.Std_G;
    Std_Impp = data.Std_Impp;

end

%% =========================================================
% NORMALIZACION
% ==========================================================
% La red fue entrenada con:
%   x1 = T normalizada
%   x2 = G normalizada
%
% Por eso, antes de evaluar la ANN se aplica la misma
% normalización usada durante el entrenamiento.

x1 = (T - Media_T)/Std_T;
x2 = (G - Media_G)/Std_G;

%% =========================================================
% CAPA OCULTA
% ==========================================================
% Cada neurona oculta usa función logsig:
%
%   logsig(n) = 1/(1+exp(-n))

N1 = b1(1) + x1*w1(1,1) + x2*w1(1,2);
N1 = 1/(1+exp(-N1));

N2 = b1(2) + x1*w1(2,1) + x2*w1(2,2);
N2 = 1/(1+exp(-N2));

N3 = b1(3) + x1*w1(3,1) + x2*w1(3,2);
N3 = 1/(1+exp(-N3));

N4 = b1(4) + x1*w1(4,1) + x2*w1(4,2);
N4 = 1/(1+exp(-N4));

N5 = b1(5) + x1*w1(5,1) + x2*w1(5,2);
N5 = 1/(1+exp(-N5));

%% =========================================================
% CAPA DE SALIDA
% ==========================================================
% La salida de la red está normalizada.

Salida_norm = b2 + ...
              N1*w2(1,1) + ...
              N2*w2(1,2) + ...
              N3*w2(1,3) + ...
              N4*w2(1,4) + ...
              N5*w2(1,5);

%% =========================================================
% DESNORMALIZACION
% ==========================================================
% Se convierte la salida normalizada a amperes.

Impp_nom = Salida_norm*Std_Impp + Media_Impp;

%% =========================================================
% CORRECCION POR RIZO DE CORRIENTE dIL
% ==========================================================
% La ANN entrega una referencia nominal Impp_nom.
%
% dIL representa el rizo pico-a-pico de la corriente del inductor.
% Al restar dIL, la referencia se desplaza hacia abajo para evitar
% que la envolvente superior del rizo supere la corriente Impp.
%
% Esto es equivalente a:
%
%   Iref = Impp_nom - dIL
%
% Finalmente se satura a cero para evitar referencias negativas.

Impp = Impp_nom - dIL;

% Saturación inferior
Impp = max(Impp,0);

end

== matlab function S_Mod_Sim_PV_V1/Fuzzy Tsukamoto Current Controller n_mppt = 99.11%, ta(2%) = 0.12 s con Steps de Irrad Interv. 2 Seg. n_mppt = 96.74%, ta(2%) = 0.12 s con Steps de Irrad Interv. 0.5 Seg. n_mppt = 99.37%, ta(2%) = 0.12 s con Curva de Irrad Este controlador puede disminuir ta e incrementar a tr para mitigar los MP en id (impacto positivo en PQ) 5/ANN ==
  data: T input; G input; Impp output; dIL input
function Impp = ANN(T,G,dIL)

persistent w1 w2 b1 b2
persistent Media_T Media_G Media_Impp
persistent Std_T Std_G Std_Impp

if isempty(w1)

    data = load('ANN_parametros.mat');

    w1 = data.w1;
    w2 = data.w2;

    b1 = data.b1;
    b2 = data.b2;

    Media_T = data.Media_T;
    Media_G = data.Media_G;
    Media_Impp = data.Media_Impp;

    Std_T = data.Std_T;
    Std_G = data.Std_G;
    Std_Impp = data.Std_Impp;

end

%% =========================================================
% NORMALIZACION
% ==========================================================
% La red fue entrenada con:
%   x1 = T normalizada
%   x2 = G normalizada
%
% Por eso, antes de evaluar la ANN se aplica la misma
% normalización usada durante el entrenamiento.

x1 = (T - Media_T)/Std_T;
x2 = (G - Media_G)/Std_G;

%% =========================================================
% CAPA OCULTA
% ==========================================================
% Cada neurona oculta usa función logsig:
%
%   logsig(n) = 1/(1+exp(-n))

N1 = b1(1) + x1*w1(1,1) + x2*w1(1,2);
N1 = 1/(1+exp(-N1));

N2 = b1(2) + x1*w1(2,1) + x2*w1(2,2);
N2 = 1/(1+exp(-N2));

N3 = b1(3) + x1*w1(3,1) + x2*w1(3,2);
N3 = 1/(1+exp(-N3));

N4 = b1(4) + x1*w1(4,1) + x2*w1(4,2);
N4 = 1/(1+exp(-N4));

N5 = b1(5) + x1*w1(5,1) + x2*w1(5,2);
N5 = 1/(1+exp(-N5));

%% =========================================================
% CAPA DE SALIDA
% ==========================================================
% La salida de la red está normalizada.

Salida_norm = b2 + ...
              N1*w2(1,1) + ...
              N2*w2(1,2) + ...
              N3*w2(1,3) + ...
              N4*w2(1,4) + ...
              N5*w2(1,5);

%% =========================================================
% DESNORMALIZACION
% ==========================================================
% Se convierte la salida normalizada a amperes.

Impp_nom = Salida_norm*Std_Impp + Media_Impp;

%% =========================================================
% CORRECCION POR RIZO DE CORRIENTE dIL
% ==========================================================
% La ANN entrega una referencia nominal Impp_nom.
%
% dIL representa el rizo pico-a-pico de la corriente del inductor.
% Al restar dIL, la referencia se desplaza hacia abajo para evitar
% que la envolvente superior del rizo supere la corriente Impp.
%
% Esto es equivalente a:
%
%   Iref = Impp_nom - dIL
%
% Finalmente se satura a cero para evitar referencias negativas.

Impp = Impp_nom - dIL;

% Saturación inferior
Impp = max(Impp,0);

end

== matlab function S_Mod_Sim_PV_V1/Fuzzy Tsukamoto Current Controller n_mppt = 99.11%, ta(2%) = 0.12 s con Steps de Irrad Interv. 2 Seg. n_mppt = 96.74%, ta(2%) = 0.12 s con Steps de Irrad Interv. 0.5 Seg. n_mppt = 99.37%, ta(2%) = 0.12 s con Curva de Irrad Este controlador puede disminuir ta e incrementar a tr para mitigar los MP en id (impacto positivo en PQ) 6/ANN ==
  data: T input; G input; Impp output; dIL input
function Impp = ANN(T,G,dIL)

persistent w1 w2 b1 b2
persistent Media_T Media_G Media_Impp
persistent Std_T Std_G Std_Impp

if isempty(w1)

    data = load('ANN_parametros.mat');

    w1 = data.w1;
    w2 = data.w2;

    b1 = data.b1;
    b2 = data.b2;

    Media_T = data.Media_T;
    Media_G = data.Media_G;
    Media_Impp = data.Media_Impp;

    Std_T = data.Std_T;
    Std_G = data.Std_G;
    Std_Impp = data.Std_Impp;

end

%% =========================================================
% NORMALIZACION
% ==========================================================
% La red fue entrenada con:
%   x1 = T normalizada
%   x2 = G normalizada
%
% Por eso, antes de evaluar la ANN se aplica la misma
% normalización usada durante el entrenamiento.

x1 = (T - Media_T)/Std_T;
x2 = (G - Media_G)/Std_G;

%% =========================================================
% CAPA OCULTA
% ==========================================================
% Cada neurona oculta usa función logsig:
%
%   logsig(n) = 1/(1+exp(-n))

N1 = b1(1) + x1*w1(1,1) + x2*w1(1,2);
N1 = 1/(1+exp(-N1));

N2 = b1(2) + x1*w1(2,1) + x2*w1(2,2);
N2 = 1/(1+exp(-N2));

N3 = b1(3) + x1*w1(3,1) + x2*w1(3,2);
N3 = 1/(1+exp(-N3));

N4 = b1(4) + x1*w1(4,1) + x2*w1(4,2);
N4 = 1/(1+exp(-N4));

N5 = b1(5) + x1*w1(5,1) + x2*w1(5,2);
N5 = 1/(1+exp(-N5));

%% =========================================================
% CAPA DE SALIDA
% ==========================================================
% La salida de la red está normalizada.

Salida_norm = b2 + ...
              N1*w2(1,1) + ...
              N2*w2(1,2) + ...
              N3*w2(1,3) + ...
              N4*w2(1,4) + ...
              N5*w2(1,5);

%% =========================================================
% DESNORMALIZACION
% ==========================================================
% Se convierte la salida normalizada a amperes.

Impp_nom = Salida_norm*Std_Impp + Media_Impp;

%% =========================================================
% CORRECCION POR RIZO DE CORRIENTE dIL
% ==========================================================
% La ANN entrega una referencia nominal Impp_nom.
%
% dIL representa el rizo pico-a-pico de la corriente del inductor.
% Al restar dIL, la referencia se desplaza hacia abajo para evitar
% que la envolvente superior del rizo supere la corriente Impp.
%
% Esto es equivalente a:
%
%   Iref = Impp_nom - dIL
%
% Finalmente se satura a cero para evitar referencias negativas.

Impp = Impp_nom - dIL;

% Saturación inferior
Impp = max(Impp,0);

end

== matlab function S_Mod_Sim_PV_V1/Mediciones A/Subsystem12/MATLAB Function ==
  data: efficiency output; Pmpp input; Pactual input; time input; t_start input; t_end input

function efficiency = n_mppt(Pmpp, Pactual, time, t_start, t_end)
%#codegen
% Calcula la eficiencia acumulada de un MPPT en porcentaje
% limitando Pactual para que no exceda Pmpp.
% Acumula solo dentro del intervalo de tiempo [t_start, t_end].
%
% Entradas:
%   Pmpp     : potencia teórica máxima (kW)
%   Pactual  : potencia medida real (kW)
%   time     : tiempo actual (segundos)
%   t_start  : inicio de acumulación
%   t_end    : fin de acumulación
%
% Salida:
%   efficiency : eficiencia acumulada (%), limitada a 100

% Variables persistentes
persistent total_Pmpp total_Pactual started

% Inicialización al primer uso
if isempty(total_Pmpp)
    total_Pmpp = 0;
    total_Pactual = 0;
    started = false;
end

% Acumular solo dentro del intervalo [t_start, t_end]
if time >= t_start && time <= t_end
    if ~started
        started = true;
    end

    % Limitar Pactual para evitar que exceda Pmpp
    %Pactual_limited = min(Pactual, Pmpp);
     
    % No Limitar Pactual 
    Pactual_limited = Pactual;

    % Acumulación
    total_Pmpp = total_Pmpp + Pmpp;
    total_Pactual = total_Pactual + Pactual_limited;
end

% Cálculo de eficiencia acumulada
if total_Pmpp < 1e-6
    efficiency = 0;
else
    efficiency = min((total_Pactual / total_Pmpp) * 100, 100);
end
end
